simulink subsystem "sensores"  (R2023b)
settings: Solver=VariableStepAuto  StartTime=0.0  StopTime=10.0  RelTol=1e-3
libraries: arduinolib x2
settings Model: Creator=Usuario_UMA  LastModifiedBy=Carlos

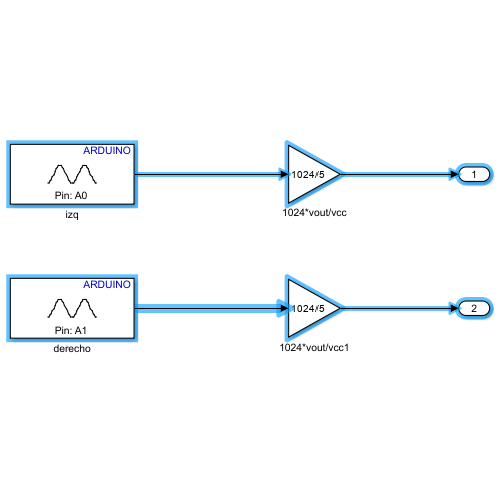
[thumbnail: Simulink's stored preview of the top-level diagram]
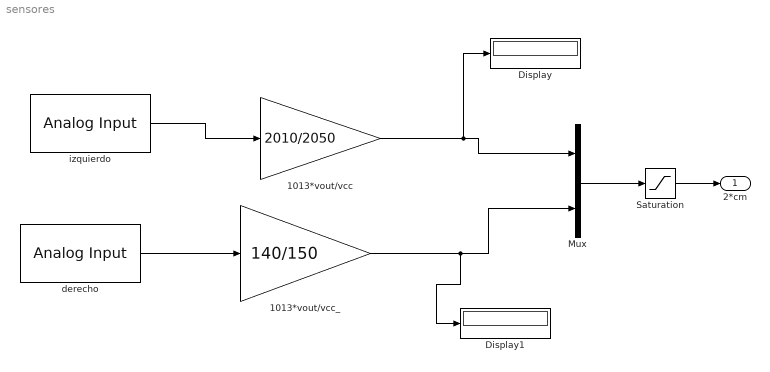
== system sensores ==
  1013*vout/vcc : Gain  Gain=2010/2050
  1013*vout/vcc_ : Gain  Gain=140/150
  Display : Display
  Display1 : Display
  Mux : Mux  Inputs=2
  Saturation : Saturate  UpperLimit=300  LowerLimit=0
  derecho : arduinolib/Analog Input  pinNumber=1  ReadResultsOnly=off  ConversionTriggerSource=Software  ExternalTriggerType=uint32( 0 )  OutputDataType=uint16  EnableConversionCompleteNotify=off  EnableOuputStatus=off  SampleTime=0.01  blockPlatform=arduino
  izquierdo : arduinolib/Analog Input  pinNumber=0  ReadResultsOnly=off  ConversionTriggerSource=Software  ExternalTriggerType=uint32( 0 )  OutputDataType=uint16  EnableConversionCompleteNotify=off  EnableOuputStatus=off  SampleTime=0.01  blockPlatform=arduino
  2*cm : Outport
  wires:
  derecho/1 -> 1013*vout/vcc_/1
  izquierdo/1 -> 1013*vout/vcc/1
  1013*vout/vcc_/1 -> Mux/2, Display1/1
  1013*vout/vcc/1 -> Mux/1, Display/1
  Mux/1 -> Saturation/1
  Saturation/1 -> 2*cm/1
